simulink subsystem "FOCCurrentControl"  (R2023b)
settings: Solver=VariableStepAuto  StartTime=0.0  StopTime=10.0  RelTol=1e-3
undefined symbols (not defined in the file): ControlCurrentPID_I, ControlCurrentPID_P, SimulationElectrical_Timestep
libraries: mcbfoclib x1
settings Model: Creator=rodri  LastModifiedBy=rodri

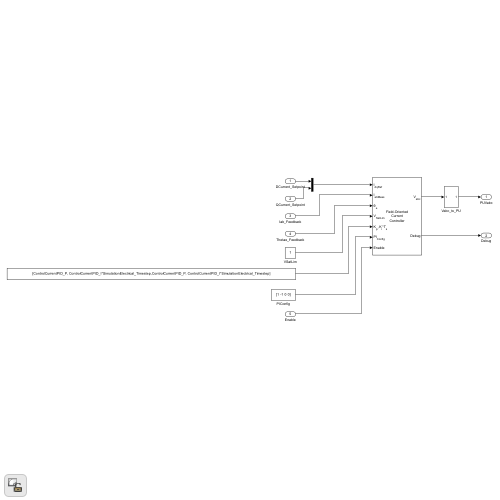
[thumbnail: Simulink's stored preview of the top-level diagram]
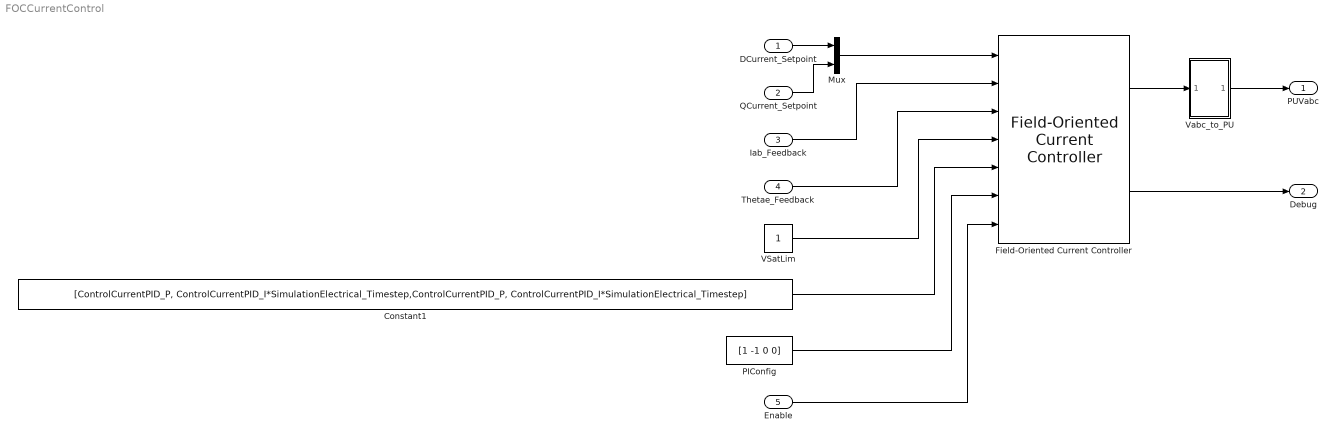
== system FOCCurrentControl ==
  DCurrent_Setpoint : Inport
  QCurrent_Setpoint : Inport  Port=2
  Iab_Feedback : Inport  Port=3
  Thetae_Feedback : Inport  Port=4
  Enable : Inport  Port=5
  Constant1 : Constant  Value=[ControlCurrentPID_P, ControlCurrentPID_I*SimulationElectrical_Timestep,ControlCurrentPID_P, ControlCurrentPID_I*SimulationElectrical_Timestep]  VectorParams1D=off  OutDataTypeStr=single
  Field-Oriented Current Controller : mcbfoclib/Field-Oriented Current Controller  AngleUnit=Radians  NumberOfLUTPoints=1024  AxisAlignment=D-axis  SaturationMethod=D-Q equivalence  PWMMethod=SVM: space vector modulation
      settings: LibrarySourceBlock=mcblib/Controls/Controllers/Field-Oriented Current Controller
  Mux : Mux  Inputs=2
  PIConfig : Constant  Value=[1 -1 0 0]  OutDataTypeStr=single
  VSatLim : Constant  OutDataTypeStr=single
  Vabc_to_PU : Subsystem
  PUVabc : Outport
  Debug : Outport  Port=2
  wires:
  Iab_Feedback/1 -> Field-Oriented Current Controller/2
  Thetae_Feedback/1 -> Field-Oriented Current Controller/3
  DCurrent_Setpoint/1 -> Mux/1
  QCurrent_Setpoint/1 -> Mux/2
  Mux/1 -> Field-Oriented Current Controller/1
  VSatLim/1 -> Field-Oriented Current Controller/4
  Constant1/1 -> Field-Oriented Current Controller/5
  PIConfig/1 -> Field-Oriented Current Controller/6
  Enable/1 -> Field-Oriented Current Controller/7
  Field-Oriented Current Controller/1 -> Vabc_to_PU/1(In1)
  Vabc_to_PU/1(Out1) -> PUVabc/1
  Field-Oriented Current Controller/2 -> Debug/1

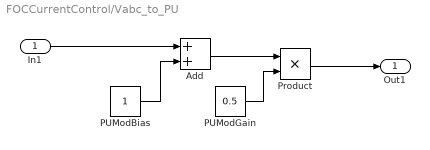
== system FOCCurrentControl/Vabc_to_PU ==
  In1 : Inport
  Add : Sum
  PUModBias : Constant
  PUModGain : Constant  Value=0.5
  Product : Product
  Out1 : Outport
  wires:
  In1/1 -> Add/1
  Product/1 -> Out1/1
  PUModGain/1 -> Product/2
  Add/1 -> Product/1
  PUModBias/1 -> Add/2
